simulink model "MPG_MG_PLL_orig"  (R2021b)
settings: Solver=VariableStepAuto  StartTime=0.0  StopTime=1  RelTol=1e-3
model workspace (MAT data in the model file):
  Ts : Simulink.Parameter (value not decoded)
  secondary_on : Simulink.Parameter (value not decoded)
values from neighbouring files (symbols this model uses):
  A = zeros(4,4)    [MPC_MG_script_raw_dmpc.m]    (also in MPG_MG_July.m = [0 1 1 1; 1 0 0 0; 1 0 0 0; 1 0 0 0]; MPG_MG_freq_script.m = ones(4) - eye(4); Script.m = [0 1 1 1 ; 1 0 1 1 ; 1 1 0 1 ; 1 1 1 0])
  C_f = 50e-6    (= 5e-05)    [Four_DG_MG_PrimaryOnlyScript.m]    (also in MPC_MG_script.m; MPC_MG_script_raw_dmpc.m; MPC_MG_secondary_script.m; MPG_MG_July.m)
  f_c = 5000    [Four_DG_MG_PrimaryOnlyScript.m]    (also in MPC_MG_script.m = 40000; MPC_MG_script_raw_dmpc.m = 40000; MPC_MG_secondary_script.m = 40000; MPG_MG_July.m = 50000)
  kL = 1e-5    (= 1e-05)    [Four_DG_MG_PrimaryOnlyScript.m]    (also in MPC_MG_script.m = 1e-08; MPC_MG_script_raw_dmpc.m = 1e-08; MPC_MG_secondary_script.m = 1e-07; MPG_MG_July.m = 1e-07)
  L_f = 1.35e-3    (= 0.00135)    [Four_DG_MG_PrimaryOnlyScript.m]    (also in MPC_MG_script.m; MPC_MG_script_raw_dmpc.m; MPC_MG_secondary_script.m; MPG_MG_July.m)
  L_in1 = 0.35e-3    (= 0.00035)    [Four_DG_MG_PrimaryOnlyScript.m]    (also in MPC_MG_script.m; MPC_MG_script_raw_dmpc.m; MPC_MG_secondary_script.m; MPG_MG_July.m)
  L_in2 = 0.35e-3    (= 0.00035)    [Four_DG_MG_PrimaryOnlyScript.m]    (also in MPC_MG_script.m; MPC_MG_script_raw_dmpc.m; MPC_MG_secondary_script.m; MPG_MG_July.m)
  L_in4 = 0.35e-3    (= 0.00035)    [Four_DG_MG_PrimaryOnlyScript.m]    (also in MPC_MG_script.m; MPC_MG_script_raw_dmpc.m; MPC_MG_secondary_script.m; MPG_MG_July.m)
  lambda1 = [30000 50000 90000 50000]'    [MPC_MG_script_raw_dmpc.m]    (also in MPG_MG_July.m = [4 4 4 4]'; MPG_MG_freq_script.m = [3 3 3 3]'; Script.m = [1 1 1 1]')
  lambda2 = [5 6 7 6]'    [MPC_MG_script_raw_dmpc.m]    (also in MPG_MG_July.m = [0.5e-2 0.5e-2 0.5e-2 0.5e-2]'; MPG_MG_freq_script.m = [1.1 1.9 1.5 1.2]'; Script.m = [0.8e-2 0.8e-2 0.8e-2 0.8e-2]')
  lambda3 = [80000 80000 900000 80000]'    [MPC_MG_script_raw_dmpc.m]    (also in MPG_MG_July.m = [1e-3 1e-3 1e-3 1e-3]'; MPG_MG_freq_script.m = [9e-4 1.2e-2 3e-3 3e-3]'; Script.m = [1.5e-3 1.5e-3 1.5e-3 1.5e-3]')
  LD_ref1 = 800e-6    (= 0.0008)    [Four_DG_MG_PrimaryOnlyScript.m]    (also in MPC_MG_script.m = 0.0003; MPC_MG_script_raw_dmpc.m = 0.0003; MPC_MG_secondary_script.m = 0.0001; MPG_MG_July.m = 0.0004)
  lo_co = 0.2    [Four_DG_MG_PrimaryOnlyScript.m]    (also in MPC_MG_script.m = 0.05; MPC_MG_script_raw_dmpc.m; MPC_MG_secondary_script.m = 0.08; MPG_MG_July.m = 0.15)
  m_p1 = 9.4e-5/droopDivide    (= 9.4e-05)    [Four_DG_MG_PrimaryOnlyScript.m]    (also in MPC_MG_script.m; MPC_MG_script_raw_dmpc.m; MPC_MG_secondary_script.m; MPG_MG_July.m)
  m_p2 = 9.4e-5/droopDivide    (= 9.4e-05)    [Four_DG_MG_PrimaryOnlyScript.m]    (also in MPC_MG_script.m; MPC_MG_script_raw_dmpc.m; MPC_MG_secondary_script.m; MPG_MG_July.m)
  m_p3 = 12.5e-5/droopDivide    (= 0.000125)    [Four_DG_MG_PrimaryOnlyScript.m]    (also in MPC_MG_script.m; MPC_MG_script_raw_dmpc.m; MPC_MG_secondary_script.m; MPG_MG_July.m)
  m_p4 = 12.5e-5/droopDivide    (= 0.000125)    [Four_DG_MG_PrimaryOnlyScript.m]    (also in MPC_MG_script.m; MPC_MG_script_raw_dmpc.m; MPC_MG_secondary_script.m; MPG_MG_July.m)
  N = 3    [MPG_MG_July.m]    (also in MPG_MG_freq_script.m = 2; Script.m = 5)
  n_q1 = 1.3e-3/droopDivide2    (= 0.00013)    [Four_DG_MG_PrimaryOnlyScript.m]    (also in MPC_MG_script.m; MPC_MG_script_raw_dmpc.m; MPC_MG_secondary_script.m; MPG_MG_July.m)
  n_q2 = 1.3e-3/droopDivide2    (= 0.00013)    [Four_DG_MG_PrimaryOnlyScript.m]    (also in MPC_MG_script.m; MPC_MG_script_raw_dmpc.m; MPC_MG_secondary_script.m; MPG_MG_July.m)
  n_q4 = 1.5e-3/droopDivide2    (= 0.00015)    [Four_DG_MG_PrimaryOnlyScript.m]    (also in MPC_MG_script.m; MPC_MG_script_raw_dmpc.m; MPC_MG_secondary_script.m; MPG_MG_July.m)
  Pmax = [45e3 45e3 37e3 37e3]'    [MPG_MG_July.m]    (also in MPG_MG_freq_script.m; Script.m)
  R_f = 0.1    [Four_DG_MG_PrimaryOnlyScript.m]    (also in MPC_MG_script.m; MPC_MG_script_raw_dmpc.m; MPC_MG_secondary_script.m; MPG_MG_July.m)
  R_in1 = 0.03    [Four_DG_MG_PrimaryOnlyScript.m]    (also in MPC_MG_script.m; MPC_MG_script_raw_dmpc.m; MPC_MG_secondary_script.m; MPG_MG_July.m)
  R_in2 = 0.03    [Four_DG_MG_PrimaryOnlyScript.m]    (also in MPC_MG_script.m; MPC_MG_script_raw_dmpc.m; MPC_MG_secondary_script.m; MPG_MG_July.m)
  R_in4 = 0.03    [Four_DG_MG_PrimaryOnlyScript.m]    (also in MPC_MG_script.m; MPC_MG_script_raw_dmpc.m; MPC_MG_secondary_script.m; MPG_MG_July.m)
  time_thresh = 0.6    [Four_DG_MG_PrimaryOnlyScript.m]    (also in MPC_MG_script_raw_dmpc.m = 1.5; MPC_MG_secondary_script.m = 2; MPG_MG_July.m = 0.5; MPG_MG_freq_script.m = 0.5)
  Ts = 10e-6    (= 1e-05)    [Four_DG_MG_PrimaryOnlyScript.m]    (also in MPC_MG_script.m; MPC_MG_script_raw_dmpc.m; MPC_MG_secondary_script.m; MPG_MG_July.m)
  Tsamp = 0.1    [MPG_MG_July.m]    (also in MPG_MG_freq_script.m; Script.m)
  V_nom = 220*sqrt(2)    [Four_DG_MG_PrimaryOnlyScript.m]    (also in MPC_MG_script.m; MPC_MG_script_raw_dmpc.m; MPC_MG_secondary_script.m; MPG_MG_July.m)
  Vdc = 600    [Four_DG_MG_PrimaryOnlyScript.m]    (also in MPC_MG_script.m; MPC_MG_script_raw_dmpc.m; MPC_MG_secondary_script.m; MPG_MG_July.m)
  w_c_high = 2*pi*50    (= 314.159265359)    [Four_DG_MG_PrimaryOnlyScript.m]    (also in MPC_MG_script.m; MPC_MG_script_raw_dmpc.m; MPC_MG_secondary_script.m; MPG_MG_July.m)
  w_nom = 2*pi*50    (= 314.159265359)    [Four_DG_MG_PrimaryOnlyScript.m]    (also in MPC_MG_script.m; MPC_MG_script_raw_dmpc.m; MPC_MG_secondary_script.m; MPG_MG_July.m)
undefined symbols (not defined in the file or in its folder): i
libraries: spsThreePhaseSeriesRLCBranchLib x18, spsabctodq0Lib x16, spsThreePhaseVIMeasurementLib x15, eeGeneralControl x15, dspswit3 x5, spsDCVoltageSourceLib x5, spsSeriesRLCBranchLib x5, spsTwoLevelConverterLib x5, slpidlib x5, spsAlphaBetaZerotodq0Lib x4, spsSecondOrderFilterLib x4, spsThreePhaseSeriesRLCLoadLib x2
(part 4 of 6)

== system MPG_MG_PLL_orig/Voltage Source Inverter 3/Pll1phase/TienXuly ==
  v : Inport
  Gain : Gain  Gain=k
  Integrator : Integrator
  Integrator1 : Integrator
  Locthongthap : TransferFcn  Denominator=[1/fc2 1]
  Mux : Mux  Inputs=2
  Product : Product  RndMeth=Zero
  Product1 : Product  RndMeth=Zero
  Sum : Sum  Inputs=|+-
  Sum1 : Sum  Inputs=|+-
  Sum2 : Sum  Inputs=|+-
  v'-qv' : Scope
  wloc : Constant  Value=fc1*2*pi
  v' : Outport  VectorParamsAs1DForOutWhenUnconnected=off
  v'q : Outport  Port=2  VectorParamsAs1DForOutWhenUnconnected=off
  wires:
  Sum/1 -> Gain/1
  Gain/1 -> Sum1/1, Locthongthap/1
  Sum1/1 -> Product/1
  wloc/1 -> Product/2, Product1/1
  Product/1 -> Integrator/1
  Product1/1 -> Integrator1/1
  Integrator1/1 -> Sum1/2, Sum2/1
  Integrator/1 -> Product1/2, Sum/2, Mux/2, v'/1
  Locthongthap/1 -> Sum2/2
  v/1 -> Sum/1
  Sum2/1 -> v'q/1, Mux/1
  Mux/1 -> v'-qv'/1

== system MPG_MG_PLL_orig/Voltage Source Inverter 3/Pll1phase/apha-beta=>dq ==
  Theta : Inport
  Uapha : Inport  Port=2
  Ubeta : Inport  Port=3
  Mux : Mux  Inputs=3
  Tinhvd : Fcn  Expr=(u[2]*cos(u[1])+u[3]*sin(u[1]))
  Tinhvq : Fcn  Expr=(-u[2]*sin(u[1])+u[3]*cos(u[1]))
  vq : Outport  VectorParamsAs1DForOutWhenUnconnected=off
  vd : Outport  Port=2  VectorParamsAs1DForOutWhenUnconnected=off
  wires:
  Theta/1 -> Mux/1
  Uapha/1 -> Mux/2
  Ubeta/1 -> Mux/3
  Mux/1 -> Tinhvd/1, Tinhvq/1
  Tinhvd/1 -> vd/1
  Tinhvq/1 -> vq/1

== system MPG_MG_PLL_orig/Voltage Source Inverter 3/dq converter/Subsystem ==
  abc : Inport
  wt : Inport  Port=2
  Demux : Demux  Outputs=3
  abc to dq0 : spsabctodq0Lib/abc to dq0  Alignment=90 degrees behind phase A axis
  Out1 : Outport
  Out2 : Outport  Port=2
  wires:
  Demux/1 -> Out1/1
  abc to dq0/1 -> Demux/1
  wt/1 -> abc to dq0/2
  Demux/2 -> Out2/1
  abc/1 -> abc to dq0/1

== system MPG_MG_PLL_orig/Voltage Source Inverter 3/dq converter/Subsystem1 ==
  abc : Inport
  wt : Inport  Port=2
  Demux : Demux  Outputs=3
  abc to dq0 : spsabctodq0Lib/abc to dq0  Alignment=90 degrees behind phase A axis
  Out1 : Outport
  Out2 : Outport  Port=2
  wires:
  Demux/1 -> Out1/1
  abc to dq0/1 -> Demux/1
  wt/1 -> abc to dq0/2
  Demux/2 -> Out2/1
  abc/1 -> abc to dq0/1

== system MPG_MG_PLL_orig/Voltage Source Inverter 3/dq converter/Subsystem2 ==
  abc : Inport
  wt : Inport  Port=2
  Demux : Demux  Outputs=3
  abc to dq0 : spsabctodq0Lib/abc to dq0  Alignment=90 degrees behind phase A axis
  Out1 : Outport
  Out2 : Outport  Port=2
  wires:
  Demux/1 -> Out1/1
  abc to dq0/1 -> Demux/1
  wt/1 -> abc to dq0/2
  Demux/2 -> Out2/1
  abc/1 -> abc to dq0/1

== system MPG_MG_PLL_orig/Voltage Source Inverter 4/CDSC-PLL/DSC16 ==
  Alpha : Inport
  Beta : Inport  Port=2
  DSC_Beta : Subsystem
  DSC_alpha : Subsystem
  DSC2_alp : Outport  VectorParamsAs1DForOutWhenUnconnected=off
  DSC2_Bet : Outport  Port=2  VectorParamsAs1DForOutWhenUnconnected=off
  wires:
  Beta/1 -> DSC_Beta/2(Beta), DSC_alpha/2(Beta)
  Alpha/1 -> DSC_alpha/1(Alpha), DSC_Beta/1(Alpha)
  DSC_Beta/1(Out) -> DSC2_Bet/1
  DSC_alpha/1(Out) -> DSC2_alp/1

== system MPG_MG_PLL_orig/Voltage Source Inverter 4/CDSC-PLL/DSC2 ==
  Alpha : Inport
  Beta : Inport  Port=2
  DSC_Beta : Subsystem
  DSC_alpha : Subsystem
  DSC2_alp : Outport  VectorParamsAs1DForOutWhenUnconnected=off
  DSC2_Bet : Outport  Port=2  VectorParamsAs1DForOutWhenUnconnected=off
  wires:
  DSC_alpha/1(Out) -> DSC2_alp/1
  DSC_Beta/1(Out) -> DSC2_Bet/1
  Alpha/1 -> DSC_Beta/1(Alpha), DSC_alpha/1(Alpha)
  Beta/1 -> DSC_alpha/2(Beta), DSC_Beta/2(Beta)

== system MPG_MG_PLL_orig/Voltage Source Inverter 4/CDSC-PLL/DSC4 ==
  Alpha : Inport
  Beta : Inport  Port=2
  DSC_Beta : Subsystem
  DSC_alpha : Subsystem
  DSC2_alp : Outport  VectorParamsAs1DForOutWhenUnconnected=off
  DSC2_Bet : Outport  Port=2  VectorParamsAs1DForOutWhenUnconnected=off
  wires:
  Beta/1 -> DSC_Beta/2(Beta), DSC_alpha/2(Beta)
  Alpha/1 -> DSC_alpha/1(Alpha), DSC_Beta/1(Alpha)
  DSC_Beta/1(Out) -> DSC2_Bet/1
  DSC_alpha/1(Out) -> DSC2_alp/1

== system MPG_MG_PLL_orig/Voltage Source Inverter 4/CDSC-PLL/DSC8 ==
  Alpha : Inport
  Beta : Inport  Port=2
  DSC_Beta : Subsystem
  DSC_alpha : Subsystem
  DSC2_alp : Outport  VectorParamsAs1DForOutWhenUnconnected=off
  DSC2_Bet : Outport  Port=2  VectorParamsAs1DForOutWhenUnconnected=off
  wires:
  DSC_alpha/1(Out) -> DSC2_alp/1
  DSC_Beta/1(Out) -> DSC2_Bet/1
  Alpha/1 -> DSC_Beta/1(Alpha), DSC_alpha/1(Alpha)
  Beta/1 -> DSC_alpha/2(Beta), DSC_Beta/2(Beta)

== system MPG_MG_PLL_orig/Voltage Source Inverter 4/CDSC-PLL/SRF-PLL1 ==
  al-be-0 : Inport
  1/2/pi : Gain  Gain=1/(2*pi)
  2 : Constant  Value=2*pi
  3 : Constant  Value=0
  Al_Be_0 to dq0 : Subsystem
      mask Display:
      | plot([0 1], [0,1])
      | port_label('input', 1, '\alpha\beta0','texmode','on')
      | port_label('input', 2, 'wt')
      | port_label('output', 1, 'dq0')
  Integrator : Integrator
  Math Function : Math  Operator=mod  SignedPower=on  SaturateOnIntegerOverflow=on
  "PI " : slpidlib/PID Controller  Controller=PI  Form=Parallel  TimeDomain=Continuous-time  UseExternalTs=off  SampleTime=100e-6  IntegratorMethod=Forward Euler  FilterMethod=Forward Euler  ControllerParametersSource=internal  P=10  I=30  D=0  UseFilter=on  N=100  TunerSelectOption=Transfer Function Based (PID Tuner App)  InitialConditionSource=internal  InitialConditionForIntegrator=0  InitialConditionForFilter=0  DifferentiatorICPrevScaledInput=0  ExternalReset=none  TrackingMode=off  Kt=1  LimitOutput=off  SatLimitsSource=internal  UpperSaturationLimit=inf  LowerSaturationLimit=-inf  LinearizeAsGain=on  AntiWindupMode=none  Kb=1  POutMin=[]  POutMax=[]  IOutMin=[]  IOutMax=[]  DOutMin=[]  DOutMax=[]  NOutMin=[]  NOutMax=[]  SumOutMin=[]  SumOutMax=[]  SaturationOutMin=[]  SaturationOutMax=[]  PParamMin=[]  PParamMax=[]  IParamMin=[]  IParamMax=[]  DParamMin=[]  DParamMax=[]  NParamMin=[]  NParamMax=[]  KbParamMin=[]  KbParamMax=[]  KtParamMin=[]  KtParamMax=[]  KbOutMin=[]  KbOutMax=[]  KtOutMin=[]  KtOutMax=[]  IntegratorOutMin=[]  IntegratorOutMax=[]  FilterOutMin=[]  FilterOutMax=[]  SumI1OutMin=[]  SumI1OutMax=[]  SumI2OutMin=[]  SumI2OutMax=[]  SumI3OutMin=[]  SumI3OutMax=[]  SumI4OutMin=[]  SumI4OutMax=[]  SumDOutMin=[]  SumDOutMax=[]  DifferentiatorOutMin=[]  DifferentiatorOutMax=[]  FilterDiffOutCoefMin=[]  FilterDiffOutCoefMax=[]  ReciprocalOutMin=[]  ReciprocalOutMax=[]  SumDenOutMin=[]  SumDenOutMax=[]  SumNumOutMin=[]  SumNumOutMax=[]  DivideOutMin=[]  DivideOutMax=[]  UdiffTsProdOutMin=[]  UdiffTsProdOutMax=[]  NTsProdOutMin=[]  NTsProdOutMax=[]  UintegralTsProdOutMin=[]  UintegralTsProdOutMax=[]  UngainTsProdOutMin=[]  UngainTsProdOutMax=[]  IntegratorContinuousStateAttributes=''  IntegratorStateMustResolveToSignalObject=off  IntegratorRTWStateStorageClass=Auto  FilterContinuousStateAttributes=''  FilterStateMustResolveToSignalObject=off  FilterRTWStateStorageClass=Auto  ParallelPVariant=InternalParameters  IdealPVariant=Disabled  IVariant=InternalParameters  DVariant=Disabled  IntegratorVariant=Continuous  SatVariant=Disabled  AWVariant=Passthrough  PCopyVariant=Disabled  TRVariant=Disabled  FdbkBlocksVariant=Forward  IdealPFdbkVariant=Disabled  SatFdbkVariant=Disabled  DerivativeFilterVariant=Disabled  NVariant=Disabled  NCopyVariant=Disabled_SignalSpec  FilterICVariant=Disabled  IntegratorICVariant=InternalICs  ExternalResetVariant=Disabled  TRSumVariant=Passthrough  SumFdbkVariant=Disabled  SumVariant=Sum_PI  TsampFilterVariant=InternalTs  TsampNgainVariant=Passthrough  TsampIntegralVariant=Passthrough  ExternalSaturationOutDataTypeStr=Inherit: Same as second input
  Scope2 : Scope  NumInputPorts=2
  Second-Order Filter : spsSecondOrderFilterLib/Second-Order Filter  FilterType=Lowpass  Fo=5  Zeta=0.707  Ts=0  Initialize=off  Vac_Init="[0,  0,  50]"  Vdc_Init=0  PlotResponse=off  FreqRange=[0, 500, 1]
      settings: SourceProductBaseCode=PS
  Selector : Selector  InputPortWidth=3  IndexOptions=Index vector (dialog)  Indices=1  OutputSizes=1
  Sum1 : Sum  Inputs=|++
  Sum2 : Sum  Inputs=|+-
  w : Constant  Value=100*pi
  f : Outport  VectorParamsAs1DForOutWhenUnconnected=off
  wt : Outport  Port=2  VectorParamsAs1DForOutWhenUnconnected=off
  wires:
  1/2/pi/1 -> Second-Order Filter/1, Scope2/2
  Math Function/1 -> Al_Be_0 to dq0/2(wt), wt/1
  Integrator/1 -> Math Function/1
  2/1 -> Math Function/2
  Sum1/1 -> Integrator/1, 1/2/pi/1
  w/1 -> Sum1/2
  "PI "/1 -> Sum1/1
  Sum2/1 -> "PI "/1
  al-be-0/1 -> Al_Be_0 to dq0/1(Al_Be_0)
  3/1 -> Sum2/2
  Al_Be_0 to dq0/1(dq0) -> Selector/1
  Selector/1 -> Sum2/1, Scope2/1
  Second-Order Filter/1 -> f/1

== system MPG_MG_PLL_orig/Voltage Source Inverter 4/CDSC-PLL/abc to alpha-beta-Zero ==
  abc : Inport
  Gain1 : Gain  Gain=(2/3)  SaturateOnIntegerOverflow=on  OutDataTypeStr=Inherit: Same as input  ParamDataTypeStr=Inherit: Same as input
  Gain3 : Gain  Gain="[ 1   -1/2   -1/2; 0   sqrt(3)/2   -sqrt(3)/2; 1/(2)  1/(2)  1/(2) ]"  Multiplication=Matrix(K*u) (u vector)  SaturateOnIntegerOverflow=on  OutDataTypeStr=Inherit: Same as input  ParamDataTypeStr=Inherit: Same as input
  al_be_0 : Outport  VectorParamsAs1DForOutWhenUnconnected=off
  wires:
  Gain3/1 -> Gain1/1
  Gain1/1 -> al_be_0/1
  abc/1 -> Gain3/1

== system MPG_MG_PLL_orig/Voltage Source Inverter 4/dq converter/Subsystem ==
  abc : Inport
  wt : Inport  Port=2
  Demux : Demux  Outputs=3
  abc to dq0 : spsabctodq0Lib/abc to dq0  Alignment=90 degrees behind phase A axis
  Out1 : Outport
  Out2 : Outport  Port=2
  wires:
  Demux/1 -> Out1/1
  abc to dq0/1 -> Demux/1
  wt/1 -> abc to dq0/2
  Demux/2 -> Out2/1
  abc/1 -> abc to dq0/1

== system MPG_MG_PLL_orig/Voltage Source Inverter 4/dq converter/Subsystem1 ==
  abc : Inport
  wt : Inport  Port=2
  Demux : Demux  Outputs=3
  abc to dq0 : spsabctodq0Lib/abc to dq0  Alignment=90 degrees behind phase A axis
  Out1 : Outport
  Out2 : Outport  Port=2
  wires:
  Demux/1 -> Out1/1
  abc to dq0/1 -> Demux/1
  wt/1 -> abc to dq0/2
  Demux/2 -> Out2/1
  abc/1 -> abc to dq0/1

== system MPG_MG_PLL_orig/Voltage Source Inverter 4/dq converter/Subsystem2 ==
  abc : Inport
  wt : Inport  Port=2
  Demux : Demux  Outputs=3
  abc to dq0 : spsabctodq0Lib/abc to dq0  Alignment=90 degrees behind phase A axis
  Out1 : Outport
  Out2 : Outport  Port=2
  wires:
  Demux/1 -> Out1/1
  abc to dq0/1 -> Demux/1
  wt/1 -> abc to dq0/2
  Demux/2 -> Out2/1
  abc/1 -> abc to dq0/1

== system MPG_MG_PLL_orig/Voltage Source Inverter 5/CDSC-PLL/DSC16 ==
  Alpha : Inport
  Beta : Inport  Port=2
  DSC_Beta : Subsystem
  DSC_alpha : Subsystem
  DSC2_alp : Outport  VectorParamsAs1DForOutWhenUnconnected=off
  DSC2_Bet : Outport  Port=2  VectorParamsAs1DForOutWhenUnconnected=off
  wires:
  Beta/1 -> DSC_Beta/2(Beta), DSC_alpha/2(Beta)
  Alpha/1 -> DSC_alpha/1(Alpha), DSC_Beta/1(Alpha)
  DSC_Beta/1(Out) -> DSC2_Bet/1
  DSC_alpha/1(Out) -> DSC2_alp/1

== system MPG_MG_PLL_orig/Voltage Source Inverter 5/CDSC-PLL/DSC2 ==
  Alpha : Inport
  Beta : Inport  Port=2
  DSC_Beta : Subsystem
  DSC_alpha : Subsystem
  DSC2_alp : Outport  VectorParamsAs1DForOutWhenUnconnected=off
  DSC2_Bet : Outport  Port=2  VectorParamsAs1DForOutWhenUnconnected=off
  wires:
  DSC_alpha/1(Out) -> DSC2_alp/1
  DSC_Beta/1(Out) -> DSC2_Bet/1
  Alpha/1 -> DSC_Beta/1(Alpha), DSC_alpha/1(Alpha)
  Beta/1 -> DSC_alpha/2(Beta), DSC_Beta/2(Beta)

== system MPG_MG_PLL_orig/Voltage Source Inverter 5/CDSC-PLL/DSC4 ==
  Alpha : Inport
  Beta : Inport  Port=2
  DSC_Beta : Subsystem
  DSC_alpha : Subsystem
  DSC2_alp : Outport  VectorParamsAs1DForOutWhenUnconnected=off
  DSC2_Bet : Outport  Port=2  VectorParamsAs1DForOutWhenUnconnected=off
  wires:
  Beta/1 -> DSC_Beta/2(Beta), DSC_alpha/2(Beta)
  Alpha/1 -> DSC_alpha/1(Alpha), DSC_Beta/1(Alpha)
  DSC_Beta/1(Out) -> DSC2_Bet/1
  DSC_alpha/1(Out) -> DSC2_alp/1

== system MPG_MG_PLL_orig/Voltage Source Inverter 5/CDSC-PLL/DSC8 ==
  Alpha : Inport
  Beta : Inport  Port=2
  DSC_Beta : Subsystem
  DSC_alpha : Subsystem
  DSC2_alp : Outport  VectorParamsAs1DForOutWhenUnconnected=off
  DSC2_Bet : Outport  Port=2  VectorParamsAs1DForOutWhenUnconnected=off
  wires:
  DSC_alpha/1(Out) -> DSC2_alp/1
  DSC_Beta/1(Out) -> DSC2_Bet/1
  Alpha/1 -> DSC_Beta/1(Alpha), DSC_alpha/1(Alpha)
  Beta/1 -> DSC_alpha/2(Beta), DSC_Beta/2(Beta)

== system MPG_MG_PLL_orig/Voltage Source Inverter 5/CDSC-PLL/SRF-PLL1 ==
  al-be-0 : Inport
  1/2/pi : Gain  Gain=1/(2*pi)
  2 : Constant  Value=2*pi
  3 : Constant  Value=0
  Al_Be_0 to dq0 : Subsystem
      mask Display:
      | plot([0 1], [0,1])
      | port_label('input', 1, '\alpha\beta0','texmode','on')
      | port_label('input', 2, 'wt')
      | port_label('output', 1, 'dq0')
  Integrator : Integrator
  Math Function : Math  Operator=mod  SignedPower=on  SaturateOnIntegerOverflow=on
  "PI " : slpidlib/PID Controller  Controller=PI  Form=Parallel  TimeDomain=Continuous-time  UseExternalTs=off  SampleTime=100e-6  IntegratorMethod=Forward Euler  FilterMethod=Forward Euler  ControllerParametersSource=internal  P=10  I=30  D=0  UseFilter=on  N=100  TunerSelectOption=Transfer Function Based (PID Tuner App)  InitialConditionSource=internal  InitialConditionForIntegrator=0  InitialConditionForFilter=0  DifferentiatorICPrevScaledInput=0  ExternalReset=none  TrackingMode=off  Kt=1  LimitOutput=off  SatLimitsSource=internal  UpperSaturationLimit=inf  LowerSaturationLimit=-inf  LinearizeAsGain=on  AntiWindupMode=none  Kb=1  POutMin=[]  POutMax=[]  IOutMin=[]  IOutMax=[]  DOutMin=[]  DOutMax=[]  NOutMin=[]  NOutMax=[]  SumOutMin=[]  SumOutMax=[]  SaturationOutMin=[]  SaturationOutMax=[]  PParamMin=[]  PParamMax=[]  IParamMin=[]  IParamMax=[]  DParamMin=[]  DParamMax=[]  NParamMin=[]  NParamMax=[]  KbParamMin=[]  KbParamMax=[]  KtParamMin=[]  KtParamMax=[]  KbOutMin=[]  KbOutMax=[]  KtOutMin=[]  KtOutMax=[]  IntegratorOutMin=[]  IntegratorOutMax=[]  FilterOutMin=[]  FilterOutMax=[]  SumI1OutMin=[]  SumI1OutMax=[]  SumI2OutMin=[]  SumI2OutMax=[]  SumI3OutMin=[]  SumI3OutMax=[]  SumI4OutMin=[]  SumI4OutMax=[]  SumDOutMin=[]  SumDOutMax=[]  DifferentiatorOutMin=[]  DifferentiatorOutMax=[]  FilterDiffOutCoefMin=[]  FilterDiffOutCoefMax=[]  ReciprocalOutMin=[]  ReciprocalOutMax=[]  SumDenOutMin=[]  SumDenOutMax=[]  SumNumOutMin=[]  SumNumOutMax=[]  DivideOutMin=[]  DivideOutMax=[]  UdiffTsProdOutMin=[]  UdiffTsProdOutMax=[]  NTsProdOutMin=[]  NTsProdOutMax=[]  UintegralTsProdOutMin=[]  UintegralTsProdOutMax=[]  UngainTsProdOutMin=[]  UngainTsProdOutMax=[]  IntegratorContinuousStateAttributes=''  IntegratorStateMustResolveToSignalObject=off  IntegratorRTWStateStorageClass=Auto  FilterContinuousStateAttributes=''  FilterStateMustResolveToSignalObject=off  FilterRTWStateStorageClass=Auto  ParallelPVariant=InternalParameters  IdealPVariant=Disabled  IVariant=InternalParameters  DVariant=Disabled  IntegratorVariant=Continuous  SatVariant=Disabled  AWVariant=Passthrough  PCopyVariant=Disabled  TRVariant=Disabled  FdbkBlocksVariant=Forward  IdealPFdbkVariant=Disabled  SatFdbkVariant=Disabled  DerivativeFilterVariant=Disabled  NVariant=Disabled  NCopyVariant=Disabled_SignalSpec  FilterICVariant=Disabled  IntegratorICVariant=InternalICs  ExternalResetVariant=Disabled  TRSumVariant=Passthrough  SumFdbkVariant=Disabled  SumVariant=Sum_PI  TsampFilterVariant=InternalTs  TsampNgainVariant=Passthrough  TsampIntegralVariant=Passthrough  ExternalSaturationOutDataTypeStr=Inherit: Same as second input
  Scope2 : Scope  NumInputPorts=2
  Second-Order Filter : spsSecondOrderFilterLib/Second-Order Filter  FilterType=Lowpass  Fo=5  Zeta=0.707  Ts=0  Initialize=off  Vac_Init="[0,  0,  50]"  Vdc_Init=0  PlotResponse=off  FreqRange=[0, 500, 1]
      settings: SourceProductBaseCode=PS
  Selector : Selector  InputPortWidth=3  IndexOptions=Index vector (dialog)  Indices=1  OutputSizes=1
  Sum1 : Sum  Inputs=|++
  Sum2 : Sum  Inputs=|+-
  w : Constant  Value=100*pi
  f : Outport  VectorParamsAs1DForOutWhenUnconnected=off
  wt : Outport  Port=2  VectorParamsAs1DForOutWhenUnconnected=off
  wires:
  1/2/pi/1 -> Second-Order Filter/1, Scope2/2
  Math Function/1 -> Al_Be_0 to dq0/2(wt), wt/1
  Integrator/1 -> Math Function/1
  2/1 -> Math Function/2
  Sum1/1 -> Integrator/1, 1/2/pi/1
  w/1 -> Sum1/2
  "PI "/1 -> Sum1/1
  Sum2/1 -> "PI "/1
  al-be-0/1 -> Al_Be_0 to dq0/1(Al_Be_0)
  3/1 -> Sum2/2
  Al_Be_0 to dq0/1(dq0) -> Selector/1
  Selector/1 -> Sum2/1, Scope2/1
  Second-Order Filter/1 -> f/1

== system MPG_MG_PLL_orig/Voltage Source Inverter 5/CDSC-PLL/abc to alpha-beta-Zero ==
  abc : Inport
  Gain1 : Gain  Gain=(2/3)  SaturateOnIntegerOverflow=on  OutDataTypeStr=Inherit: Same as input  ParamDataTypeStr=Inherit: Same as input
  Gain3 : Gain  Gain="[ 1   -1/2   -1/2; 0   sqrt(3)/2   -sqrt(3)/2; 1/(2)  1/(2)  1/(2) ]"  Multiplication=Matrix(K*u) (u vector)  SaturateOnIntegerOverflow=on  OutDataTypeStr=Inherit: Same as input  ParamDataTypeStr=Inherit: Same as input
  al_be_0 : Outport  VectorParamsAs1DForOutWhenUnconnected=off
  wires:
  Gain3/1 -> Gain1/1
  Gain1/1 -> al_be_0/1
  abc/1 -> Gain3/1

== system MPG_MG_PLL_orig/Voltage Source Inverter 5/dq converter/Subsystem ==
  abc : Inport
  wt : Inport  Port=2
  Demux : Demux  Outputs=3
  abc to dq0 : spsabctodq0Lib/abc to dq0  Alignment=90 degrees behind phase A axis
  Out1 : Outport
  Out2 : Outport  Port=2
  wires:
  Demux/1 -> Out1/1
  abc to dq0/1 -> Demux/1
  wt/1 -> abc to dq0/2
  Demux/2 -> Out2/1
  abc/1 -> abc to dq0/1

== system MPG_MG_PLL_orig/Voltage Source Inverter 5/dq converter/Subsystem1 ==
  abc : Inport
  wt : Inport  Port=2
  Demux : Demux  Outputs=3
  abc to dq0 : spsabctodq0Lib/abc to dq0  Alignment=90 degrees behind phase A axis
  Out1 : Outport
  Out2 : Outport  Port=2
  wires:
  Demux/1 -> Out1/1
  abc to dq0/1 -> Demux/1
  wt/1 -> abc to dq0/2
  Demux/2 -> Out2/1
  abc/1 -> abc to dq0/1

== system MPG_MG_PLL_orig/Voltage Source Inverter 5/dq converter/Subsystem2 ==
  abc : Inport
  wt : Inport  Port=2
  Demux : Demux  Outputs=3
  abc to dq0 : spsabctodq0Lib/abc to dq0  Alignment=90 degrees behind phase A axis
  Out1 : Outport
  Out2 : Outport  Port=2
  wires:
  Demux/1 -> Out1/1
  abc to dq0/1 -> Demux/1
  wt/1 -> abc to dq0/2
  Demux/2 -> Out2/1
  abc/1 -> abc to dq0/1

== system MPG_MG_PLL_orig/Voltage Source Inverter 2/CDSC-PLL/DSC16/DSC_Beta ==
  Alpha : Inport
  Beta : Inport  Port=2
  Cos 2*pi/n : Subsystem
  Divide : Product  Inputs=*/
  Divide1 : Product  Inputs=*/
  Gain : Gain  Gain=1/2
  Product : Product
  Product1 : Product
  Sin 2*pi/n : Subsystem
  Sum1 : Sum  Inputs=+++
  T/n : Constant  Value=1/n
  T/n1 : Constant  Value=1/n
  Variable Transport Delay : VariableTransportDelay  VariableDelayType=Variable transport delay  MaximumDelay=10
  Variable Transport Delay1 : VariableTransportDelay  VariableDelayType=Variable transport delay  MaximumDelay=10
  Out : Outport  VectorParamsAs1DForOutWhenUnconnected=off
  wires:
  Gain/1 -> Out/1
  Sum1/1 -> Gain/1
  Beta/1 -> Variable Transport Delay/1, Sum1/1
  Alpha/1 -> Variable Transport Delay1/1
  Cos 2*pi/n/1(cos) -> Product/2
  Product/1 -> Sum1/2
  Variable Transport Delay/1 -> Product/1
  Variable Transport Delay1/1 -> Product1/1
  Product1/1 -> Sum1/3
  Sin 2*pi/n/1(sin) -> Product1/2
  T/n/1 -> Divide/1
  Divide/1 -> Variable Transport Delay/2
  [f_pll_c3] -> Divide/2
  T/n1/1 -> Divide1/1
  Divide1/1 -> Variable Transport Delay1/2
  [f_pll_c3] -> Divide1/2

== system MPG_MG_PLL_orig/Voltage Source Inverter 2/CDSC-PLL/DSC16/DSC_alpha ==
  Alpha : Inport
  Beta : Inport  Port=2
  Cos 2*pi/n : Subsystem
  Divide : Product  Inputs=*/
  Divide1 : Product  Inputs=*/
  Gain : Gain  Gain=1/2
  Product : Product
  Product1 : Product
  Sin 2*pi/n : Subsystem
  Sum1 : Sum  Inputs=++-
  T/n : Constant  Value=1/n
  T/n1 : Constant  Value=1/n
  Variable Transport Delay : VariableTransportDelay  VariableDelayType=Variable transport delay  MaximumDelay=10
  Variable Transport Delay1 : VariableTransportDelay  VariableDelayType=Variable transport delay  MaximumDelay=10
  Out : Outport  VectorParamsAs1DForOutWhenUnconnected=off
  wires:
  Sum1/1 -> Gain/1
  Gain/1 -> Out/1
  Sin 2*pi/n/1(sin) -> Product1/2
  Beta/1 -> Variable Transport Delay1/1
  Product1/1 -> Sum1/3
  Variable Transport Delay1/1 -> Product1/1
  Alpha/1 -> Variable Transport Delay/1, Sum1/1
  Variable Transport Delay/1 -> Product/1
  Product/1 -> Sum1/2
  Cos 2*pi/n/1(cos) -> Product/2
  T/n/1 -> Divide/1
  Divide/1 -> Variable Transport Delay/2
  [f_pll_c3] -> Divide/2
  T/n1/1 -> Divide1/1
  Divide1/1 -> Variable Transport Delay1/2
  [f_pll_c3] -> Divide1/2

== system MPG_MG_PLL_orig/Voltage Source Inverter 2/CDSC-PLL/DSC2/DSC_Beta ==
  Alpha : Inport
  Beta : Inport  Port=2
  Cos 2*pi/n : Subsystem
  Divide : Product  Inputs=*/
  Divide1 : Product  Inputs=*/
  Gain : Gain  Gain=1/2
  Product : Product
  Product1 : Product
  Sin 2*pi/n : Subsystem
  Sum1 : Sum  Inputs=+++
  T/n : Constant  Value=1/n
  T/n1 : Constant  Value=1/n
  Variable Transport Delay : VariableTransportDelay  VariableDelayType=Variable transport delay  MaximumDelay=10
  Variable Transport Delay1 : VariableTransportDelay  VariableDelayType=Variable transport delay  MaximumDelay=10
  Out : Outport  VectorParamsAs1DForOutWhenUnconnected=off
  wires:
  Sin 2*pi/n/1(sin) -> Product1/2
  Product1/1 -> Sum1/3
  Variable Transport Delay1/1 -> Product1/1
  Variable Transport Delay/1 -> Product/1
  Product/1 -> Sum1/2
  Cos 2*pi/n/1(cos) -> Product/2
  Alpha/1 -> Variable Transport Delay1/1
  Beta/1 -> Sum1/1, Variable Transport Delay/1
  Sum1/1 -> Gain/1
  Gain/1 -> Out/1
  T/n1/1 -> Divide/1
  Divide/1 -> Variable Transport Delay1/2
  [f_pll_c3] -> Divide/2
  T/n/1 -> Divide1/1
  Divide1/1 -> Variable Transport Delay/2
  [f_pll_c3] -> Divide1/2

== system MPG_MG_PLL_orig/Voltage Source Inverter 2/CDSC-PLL/DSC2/DSC_alpha ==
  Alpha : Inport
  Beta : Inport  Port=2
  Cos 2*pi/n : Subsystem
  Divide : Product  Inputs=*/
  Divide1 : Product  Inputs=*/
  Gain : Gain  Gain=1/2
  Product : Product
  Product1 : Product
  Sin 2*pi/n : Subsystem
  Sum1 : Sum  Inputs=++-
  T/n : Constant  Value=1/n
  T/n. : Constant  Value=1/n
  Variable Transport Delay : VariableTransportDelay  VariableDelayType=Variable transport delay  MaximumDelay=10
  Variable Transport Delay1 : VariableTransportDelay  VariableDelayType=Variable transport delay  MaximumDelay=10
  Out : Outport  VectorParamsAs1DForOutWhenUnconnected=off
  wires:
  Cos 2*pi/n/1(cos) -> Product/2
  Product/1 -> Sum1/2
  Variable Transport Delay/1 -> Product/1
  Alpha/1 -> Variable Transport Delay/1, Sum1/1
  Variable Transport Delay1/1 -> Product1/1
  Product1/1 -> Sum1/3
  Beta/1 -> Variable Transport Delay1/1
  Sin 2*pi/n/1(sin) -> Product1/2
  Gain/1 -> Out/1
  Sum1/1 -> Gain/1
  T/n/1 -> Divide/1
  Divide/1 -> Variable Transport Delay/2
  [f_pll_c3] -> Divide/2
  Divide1/1 -> Variable Transport Delay1/2
  T/n./1 -> Divide1/1
  [f_pll_c3] -> Divide1/2

== system MPG_MG_PLL_orig/Voltage Source Inverter 2/CDSC-PLL/DSC4/DSC_Beta ==
  Alpha : Inport
  Beta : Inport  Port=2
  Cos 2*pi/n : Subsystem
  Divide : Product  Inputs=*/
  Divide1 : Product  Inputs=*/
  Gain : Gain  Gain=1/2
  Product : Product
  Product1 : Product
  Sin 2*pi/n : Subsystem
  Sum1 : Sum  Inputs=+++
  T/n : Constant  Value=1/n
  T/n1 : Constant  Value=1/n
  Variable Transport Delay : VariableTransportDelay  VariableDelayType=Variable transport delay  MaximumDelay=10
  Variable Transport Delay1 : VariableTransportDelay  VariableDelayType=Variable transport delay  MaximumDelay=10
  Out : Outport  VectorParamsAs1DForOutWhenUnconnected=off
  wires:
  Gain/1 -> Out/1
  Sum1/1 -> Gain/1
  Beta/1 -> Variable Transport Delay/1, Sum1/1
  Alpha/1 -> Variable Transport Delay1/1
  Cos 2*pi/n/1(cos) -> Product/2
  Product/1 -> Sum1/2
  Variable Transport Delay/1 -> Product/1
  Variable Transport Delay1/1 -> Product1/1
  Product1/1 -> Sum1/3
  Sin 2*pi/n/1(sin) -> Product1/2
  T/n/1 -> Divide/1
  Divide/1 -> Variable Transport Delay/2
  [f_pll_c3] -> Divide/2
  T/n1/1 -> Divide1/1
  Divide1/1 -> Variable Transport Delay1/2
  [f_pll_c3] -> Divide1/2

== system MPG_MG_PLL_orig/Voltage Source Inverter 2/CDSC-PLL/DSC4/DSC_alpha ==
  Alpha : Inport
  Beta : Inport  Port=2
  Cos 2*pi/n : Subsystem
  Divide : Product  Inputs=*/
  Divide1 : Product  Inputs=*/
  Gain : Gain  Gain=1/2
  Product : Product
  Product1 : Product
  Sin 2*pi/n : Subsystem
  Sum1 : Sum  Inputs=++-
  T/n : Constant  Value=1/n
  T/n1 : Constant  Value=1/n
  Variable Transport Delay : VariableTransportDelay  VariableDelayType=Variable transport delay  MaximumDelay=10
  Variable Transport Delay1 : VariableTransportDelay  VariableDelayType=Variable transport delay  MaximumDelay=10
  Out : Outport  VectorParamsAs1DForOutWhenUnconnected=off
  wires:
  Sum1/1 -> Gain/1
  Gain/1 -> Out/1
  Sin 2*pi/n/1(sin) -> Product1/2
  Beta/1 -> Variable Transport Delay1/1
  Product1/1 -> Sum1/3
  Variable Transport Delay1/1 -> Product1/1
  Alpha/1 -> Variable Transport Delay/1, Sum1/1
  Variable Transport Delay/1 -> Product/1
  Product/1 -> Sum1/2
  Cos 2*pi/n/1(cos) -> Product/2
  T/n1/1 -> Divide/1
  Divide/1 -> Variable Transport Delay1/2
  [f_pll_c3] -> Divide/2
  T/n/1 -> Divide1/1
  Divide1/1 -> Variable Transport Delay/2
  [f_pll_c3] -> Divide1/2

== system MPG_MG_PLL_orig/Voltage Source Inverter 2/CDSC-PLL/DSC8/DSC_Beta ==
  Alpha : Inport
  Beta : Inport  Port=2
  Cos 2*pi/n : Subsystem
  Divide : Product  Inputs=*/
  Divide1 : Product  Inputs=*/
  Gain : Gain  Gain=1/2
  Product : Product
  Product1 : Product
  Sin 2*pi/n : Subsystem
  Sum1 : Sum  Inputs=+++
  T/n : Constant  Value=1/n
  T/n1 : Constant  Value=1/n
  Variable Transport Delay : VariableTransportDelay  VariableDelayType=Variable transport delay  MaximumDelay=10
  Variable Transport Delay1 : VariableTransportDelay  VariableDelayType=Variable transport delay  MaximumDelay=10
  Out : Outport  VectorParamsAs1DForOutWhenUnconnected=off
  wires:
  Sin 2*pi/n/1(sin) -> Product1/2
  Product1/1 -> Sum1/3
  Variable Transport Delay1/1 -> Product1/1
  Variable Transport Delay/1 -> Product/1
  Product/1 -> Sum1/2
  Cos 2*pi/n/1(cos) -> Product/2
  Alpha/1 -> Variable Transport Delay1/1
  Beta/1 -> Sum1/1, Variable Transport Delay/1
  Sum1/1 -> Gain/1
  Gain/1 -> Out/1
  T/n/1 -> Divide/1
  Divide/1 -> Variable Transport Delay/2
  [f_pll_c3] -> Divide/2
  T/n1/1 -> Divide1/1
  Divide1/1 -> Variable Transport Delay1/2
  [f_pll_c3] -> Divide1/2

== system MPG_MG_PLL_orig/Voltage Source Inverter 2/CDSC-PLL/DSC8/DSC_alpha ==
  Alpha : Inport
  Beta : Inport  Port=2
  Cos 2*pi/n : Subsystem
  Divide : Product  Inputs=*/
  Divide1 : Product  Inputs=*/
  Gain : Gain  Gain=1/2
  Product : Product
  Product1 : Product
  Sin 2*pi/n : Subsystem
  Sum1 : Sum  Inputs=++-
  T/n : Constant  Value=1/n
  T/n1 : Constant  Value=1/n
  Variable Transport Delay : VariableTransportDelay  VariableDelayType=Variable transport delay  MaximumDelay=10
  Variable Transport Delay1 : VariableTransportDelay  VariableDelayType=Variable transport delay  MaximumDelay=10
  Out : Outport  VectorParamsAs1DForOutWhenUnconnected=off
  wires:
  Cos 2*pi/n/1(cos) -> Product/2
  Product/1 -> Sum1/2
  Variable Transport Delay/1 -> Product/1
  Alpha/1 -> Variable Transport Delay/1, Sum1/1
  Variable Transport Delay1/1 -> Product1/1
  Product1/1 -> Sum1/3
  Beta/1 -> Variable Transport Delay1/1
  Sin 2*pi/n/1(sin) -> Product1/2
  Gain/1 -> Out/1
  Sum1/1 -> Gain/1
  T/n/1 -> Divide/1
  Divide/1 -> Variable Transport Delay/2
  [f_pll_c3] -> Divide/2
  T/n1/1 -> Divide1/1
  Divide1/1 -> Variable Transport Delay1/2
  [f_pll_c3] -> Divide1/2

== system MPG_MG_PLL_orig/Voltage Source Inverter 2/CDSC-PLL/SRF-PLL1/Al_Be_0 to dq0 ==
  Al_Be_0 : Inport
  wt : Inport  Port=2
  Fcn : Fcn  Expr=u[1]*cos(u[4]) + u[2]*sin(u[4])
  Fcn1 : Fcn  Expr=-u[1]*sin(u[4]) + u[2]*cos(u[4])
  Fcn2 : Fcn  Expr=u[3]
  Mux1 : Mux  Inputs=[3 1]
  Mux2 : Mux  Inputs=3
  dq0 : Outport  VectorParamsAs1DForOutWhenUnconnected=off
  wires:
  Mux1/1 -> Fcn/1, Fcn2/1, Fcn1/1
  Fcn1/1 -> Mux2/2
  wt/1 -> Mux1/2
  Mux2/1 -> dq0/1
  Al_Be_0/1 -> Mux1/1
  Fcn2/1 -> Mux2/3
  Fcn/1 -> Mux2/1

== system MPG_MG_PLL_orig/Voltage Source Inverter 3/CDSC-PLL/DSC16/DSC_Beta ==
  Alpha : Inport
  Beta : Inport  Port=2
  Cos 2*pi/n : Subsystem
  Divide : Product  Inputs=*/
  Divide1 : Product  Inputs=*/
  Gain : Gain  Gain=1/2
  Product : Product
  Product1 : Product
  Sin 2*pi/n : Subsystem
  Sum1 : Sum  Inputs=+++
  T/n : Constant  Value=1/n
  T/n1 : Constant  Value=1/n
  Variable Transport Delay : VariableTransportDelay  VariableDelayType=Variable transport delay  MaximumDelay=10
  Variable Transport Delay1 : VariableTransportDelay  VariableDelayType=Variable transport delay  MaximumDelay=10
  Out : Outport  VectorParamsAs1DForOutWhenUnconnected=off
  wires:
  Gain/1 -> Out/1
  Sum1/1 -> Gain/1
  Beta/1 -> Variable Transport Delay/1, Sum1/1
  Alpha/1 -> Variable Transport Delay1/1
  Cos 2*pi/n/1(cos) -> Product/2
  Product/1 -> Sum1/2
  Variable Transport Delay/1 -> Product/1
  Variable Transport Delay1/1 -> Product1/1
  Product1/1 -> Sum1/3
  Sin 2*pi/n/1(sin) -> Product1/2
  T/n/1 -> Divide/1
  Divide/1 -> Variable Transport Delay/2
  [f_pll_c3] -> Divide/2
  T/n1/1 -> Divide1/1
  Divide1/1 -> Variable Transport Delay1/2
  [f_pll_c3] -> Divide1/2

== system MPG_MG_PLL_orig/Voltage Source Inverter 3/CDSC-PLL/DSC16/DSC_alpha ==
  Alpha : Inport
  Beta : Inport  Port=2
  Cos 2*pi/n : Subsystem
  Divide : Product  Inputs=*/
  Divide1 : Product  Inputs=*/
  Gain : Gain  Gain=1/2
  Product : Product
  Product1 : Product
  Sin 2*pi/n : Subsystem
  Sum1 : Sum  Inputs=++-
  T/n : Constant  Value=1/n
  T/n1 : Constant  Value=1/n
  Variable Transport Delay : VariableTransportDelay  VariableDelayType=Variable transport delay  MaximumDelay=10
  Variable Transport Delay1 : VariableTransportDelay  VariableDelayType=Variable transport delay  MaximumDelay=10
  Out : Outport  VectorParamsAs1DForOutWhenUnconnected=off
  wires:
  Sum1/1 -> Gain/1
  Gain/1 -> Out/1
  Sin 2*pi/n/1(sin) -> Product1/2
  Beta/1 -> Variable Transport Delay1/1
  Product1/1 -> Sum1/3
  Variable Transport Delay1/1 -> Product1/1
  Alpha/1 -> Variable Transport Delay/1, Sum1/1
  Variable Transport Delay/1 -> Product/1
  Product/1 -> Sum1/2
  Cos 2*pi/n/1(cos) -> Product/2
  T/n/1 -> Divide/1
  Divide/1 -> Variable Transport Delay/2
  [f_pll_c3] -> Divide/2
  T/n1/1 -> Divide1/1
  Divide1/1 -> Variable Transport Delay1/2
  [f_pll_c3] -> Divide1/2

== system MPG_MG_PLL_orig/Voltage Source Inverter 3/CDSC-PLL/DSC2/DSC_Beta ==
  Alpha : Inport
  Beta : Inport  Port=2
  Cos 2*pi/n : Subsystem
  Divide : Product  Inputs=*/
  Divide1 : Product  Inputs=*/
  Gain : Gain  Gain=1/2
  Product : Product
  Product1 : Product
  Sin 2*pi/n : Subsystem
  Sum1 : Sum  Inputs=+++
  T/n : Constant  Value=1/n
  T/n1 : Constant  Value=1/n
  Variable Transport Delay : VariableTransportDelay  VariableDelayType=Variable transport delay  MaximumDelay=10
  Variable Transport Delay1 : VariableTransportDelay  VariableDelayType=Variable transport delay  MaximumDelay=10
  Out : Outport  VectorParamsAs1DForOutWhenUnconnected=off
  wires:
  Sin 2*pi/n/1(sin) -> Product1/2
  Product1/1 -> Sum1/3
  Variable Transport Delay1/1 -> Product1/1
  Variable Transport Delay/1 -> Product/1
  Product/1 -> Sum1/2
  Cos 2*pi/n/1(cos) -> Product/2
  Alpha/1 -> Variable Transport Delay1/1
  Beta/1 -> Sum1/1, Variable Transport Delay/1
  Sum1/1 -> Gain/1
  Gain/1 -> Out/1
  T/n1/1 -> Divide/1
  Divide/1 -> Variable Transport Delay1/2
  [f_pll_c3] -> Divide/2
  T/n/1 -> Divide1/1
  Divide1/1 -> Variable Transport Delay/2
  [f_pll_c3] -> Divide1/2

== system MPG_MG_PLL_orig/Voltage Source Inverter 3/CDSC-PLL/DSC2/DSC_alpha ==
  Alpha : Inport
  Beta : Inport  Port=2
  Cos 2*pi/n : Subsystem
  Divide : Product  Inputs=*/
  Divide1 : Product  Inputs=*/
  Gain : Gain  Gain=1/2
  Product : Product
  Product1 : Product
  Sin 2*pi/n : Subsystem
  Sum1 : Sum  Inputs=++-
  T/n : Constant  Value=1/n
  T/n. : Constant  Value=1/n
  Variable Transport Delay : VariableTransportDelay  VariableDelayType=Variable transport delay  MaximumDelay=10
  Variable Transport Delay1 : VariableTransportDelay  VariableDelayType=Variable transport delay  MaximumDelay=10
  Out : Outport  VectorParamsAs1DForOutWhenUnconnected=off
  wires:
  Cos 2*pi/n/1(cos) -> Product/2
  Product/1 -> Sum1/2
  Variable Transport Delay/1 -> Product/1
  Alpha/1 -> Variable Transport Delay/1, Sum1/1
  Variable Transport Delay1/1 -> Product1/1
  Product1/1 -> Sum1/3
  Beta/1 -> Variable Transport Delay1/1
  Sin 2*pi/n/1(sin) -> Product1/2
  Gain/1 -> Out/1
  Sum1/1 -> Gain/1
  T/n/1 -> Divide/1
  Divide/1 -> Variable Transport Delay/2
  [f_pll_c3] -> Divide/2
  Divide1/1 -> Variable Transport Delay1/2
  T/n./1 -> Divide1/1
  [f_pll_c3] -> Divide1/2

== system MPG_MG_PLL_orig/Voltage Source Inverter 3/CDSC-PLL/DSC4/DSC_Beta ==
  Alpha : Inport
  Beta : Inport  Port=2
  Cos 2*pi/n : Subsystem
  Divide : Product  Inputs=*/
  Divide1 : Product  Inputs=*/
  Gain : Gain  Gain=1/2
  Product : Product
  Product1 : Product
  Sin 2*pi/n : Subsystem
  Sum1 : Sum  Inputs=+++
  T/n : Constant  Value=1/n
  T/n1 : Constant  Value=1/n
  Variable Transport Delay : VariableTransportDelay  VariableDelayType=Variable transport delay  MaximumDelay=10
  Variable Transport Delay1 : VariableTransportDelay  VariableDelayType=Variable transport delay  MaximumDelay=10
  Out : Outport  VectorParamsAs1DForOutWhenUnconnected=off
  wires:
  Gain/1 -> Out/1
  Sum1/1 -> Gain/1
  Beta/1 -> Variable Transport Delay/1, Sum1/1
  Alpha/1 -> Variable Transport Delay1/1
  Cos 2*pi/n/1(cos) -> Product/2
  Product/1 -> Sum1/2
  Variable Transport Delay/1 -> Product/1
  Variable Transport Delay1/1 -> Product1/1
  Product1/1 -> Sum1/3
  Sin 2*pi/n/1(sin) -> Product1/2
  T/n/1 -> Divide/1
  Divide/1 -> Variable Transport Delay/2
  [f_pll_c3] -> Divide/2
  T/n1/1 -> Divide1/1
  Divide1/1 -> Variable Transport Delay1/2
  [f_pll_c3] -> Divide1/2

== system MPG_MG_PLL_orig/Voltage Source Inverter 3/CDSC-PLL/DSC4/DSC_alpha ==
  Alpha : Inport
  Beta : Inport  Port=2
  Cos 2*pi/n : Subsystem
  Divide : Product  Inputs=*/
  Divide1 : Product  Inputs=*/
  Gain : Gain  Gain=1/2
  Product : Product
  Product1 : Product
  Sin 2*pi/n : Subsystem
  Sum1 : Sum  Inputs=++-
  T/n : Constant  Value=1/n
  T/n1 : Constant  Value=1/n
  Variable Transport Delay : VariableTransportDelay  VariableDelayType=Variable transport delay  MaximumDelay=10
  Variable Transport Delay1 : VariableTransportDelay  VariableDelayType=Variable transport delay  MaximumDelay=10
  Out : Outport  VectorParamsAs1DForOutWhenUnconnected=off
  wires:
  Sum1/1 -> Gain/1
  Gain/1 -> Out/1
  Sin 2*pi/n/1(sin) -> Product1/2
  Beta/1 -> Variable Transport Delay1/1
  Product1/1 -> Sum1/3
  Variable Transport Delay1/1 -> Product1/1
  Alpha/1 -> Variable Transport Delay/1, Sum1/1
  Variable Transport Delay/1 -> Product/1
  Product/1 -> Sum1/2
  Cos 2*pi/n/1(cos) -> Product/2
  T/n1/1 -> Divide/1
  Divide/1 -> Variable Transport Delay1/2
  [f_pll_c3] -> Divide/2
  T/n/1 -> Divide1/1
  Divide1/1 -> Variable Transport Delay/2
  [f_pll_c3] -> Divide1/2

== system MPG_MG_PLL_orig/Voltage Source Inverter 3/CDSC-PLL/DSC8/DSC_Beta ==
  Alpha : Inport
  Beta : Inport  Port=2
  Cos 2*pi/n : Subsystem
  Divide : Product  Inputs=*/
  Divide1 : Product  Inputs=*/
  Gain : Gain  Gain=1/2
  Product : Product
  Product1 : Product
  Sin 2*pi/n : Subsystem
  Sum1 : Sum  Inputs=+++
  T/n : Constant  Value=1/n
  T/n1 : Constant  Value=1/n
  Variable Transport Delay : VariableTransportDelay  VariableDelayType=Variable transport delay  MaximumDelay=10
  Variable Transport Delay1 : VariableTransportDelay  VariableDelayType=Variable transport delay  MaximumDelay=10
  Out : Outport  VectorParamsAs1DForOutWhenUnconnected=off
  wires:
  Sin 2*pi/n/1(sin) -> Product1/2
  Product1/1 -> Sum1/3
  Variable Transport Delay1/1 -> Product1/1
  Variable Transport Delay/1 -> Product/1
  Product/1 -> Sum1/2
  Cos 2*pi/n/1(cos) -> Product/2
  Alpha/1 -> Variable Transport Delay1/1
  Beta/1 -> Sum1/1, Variable Transport Delay/1
  Sum1/1 -> Gain/1
  Gain/1 -> Out/1
  T/n/1 -> Divide/1
  Divide/1 -> Variable Transport Delay/2
  [f_pll_c3] -> Divide/2
  T/n1/1 -> Divide1/1
  Divide1/1 -> Variable Transport Delay1/2
  [f_pll_c3] -> Divide1/2

== system MPG_MG_PLL_orig/Voltage Source Inverter 3/CDSC-PLL/DSC8/DSC_alpha ==
  Alpha : Inport
  Beta : Inport  Port=2
  Cos 2*pi/n : Subsystem
  Divide : Product  Inputs=*/
  Divide1 : Product  Inputs=*/
  Gain : Gain  Gain=1/2
  Product : Product
  Product1 : Product
  Sin 2*pi/n : Subsystem
  Sum1 : Sum  Inputs=++-
  T/n : Constant  Value=1/n
  T/n1 : Constant  Value=1/n
  Variable Transport Delay : VariableTransportDelay  VariableDelayType=Variable transport delay  MaximumDelay=10
  Variable Transport Delay1 : VariableTransportDelay  VariableDelayType=Variable transport delay  MaximumDelay=10
  Out : Outport  VectorParamsAs1DForOutWhenUnconnected=off
  wires:
  Cos 2*pi/n/1(cos) -> Product/2
  Product/1 -> Sum1/2
  Variable Transport Delay/1 -> Product/1
  Alpha/1 -> Variable Transport Delay/1, Sum1/1
  Variable Transport Delay1/1 -> Product1/1
  Product1/1 -> Sum1/3
  Beta/1 -> Variable Transport Delay1/1
  Sin 2*pi/n/1(sin) -> Product1/2
  Gain/1 -> Out/1
  Sum1/1 -> Gain/1
  T/n/1 -> Divide/1
  Divide/1 -> Variable Transport Delay/2
  [f_pll_c3] -> Divide/2
  T/n1/1 -> Divide1/1
  Divide1/1 -> Variable Transport Delay1/2
  [f_pll_c3] -> Divide1/2

== system MPG_MG_PLL_orig/Voltage Source Inverter 3/CDSC-PLL/SRF-PLL1/Al_Be_0 to dq0 ==
  Al_Be_0 : Inport
  wt : Inport  Port=2
  Fcn : Fcn  Expr=u[1]*cos(u[4]) + u[2]*sin(u[4])
  Fcn1 : Fcn  Expr=-u[1]*sin(u[4]) + u[2]*cos(u[4])
  Fcn2 : Fcn  Expr=u[3]
  Mux1 : Mux  Inputs=[3 1]
  Mux2 : Mux  Inputs=3
  dq0 : Outport  VectorParamsAs1DForOutWhenUnconnected=off
  wires:
  Mux1/1 -> Fcn/1, Fcn2/1, Fcn1/1
  Fcn1/1 -> Mux2/2
  wt/1 -> Mux1/2
  Mux2/1 -> dq0/1
  Al_Be_0/1 -> Mux1/1
  Fcn2/1 -> Mux2/3
  Fcn/1 -> Mux2/1

== system MPG_MG_PLL_orig/Voltage Source Inverter 4/CDSC-PLL/DSC16/DSC_Beta ==
  Alpha : Inport
  Beta : Inport  Port=2
  Cos 2*pi/n : Subsystem
  Divide : Product  Inputs=*/
  Divide1 : Product  Inputs=*/
  Gain : Gain  Gain=1/2
  Product : Product
  Product1 : Product
  Sin 2*pi/n : Subsystem
  Sum1 : Sum  Inputs=+++
  T/n : Constant  Value=1/n
  T/n1 : Constant  Value=1/n
  Variable Transport Delay : VariableTransportDelay  VariableDelayType=Variable transport delay  MaximumDelay=10
  Variable Transport Delay1 : VariableTransportDelay  VariableDelayType=Variable transport delay  MaximumDelay=10
  Out : Outport  VectorParamsAs1DForOutWhenUnconnected=off
  wires:
  Gain/1 -> Out/1
  Sum1/1 -> Gain/1
  Beta/1 -> Variable Transport Delay/1, Sum1/1
  Alpha/1 -> Variable Transport Delay1/1
  Cos 2*pi/n/1(cos) -> Product/2
  Product/1 -> Sum1/2
  Variable Transport Delay/1 -> Product/1
  Variable Transport Delay1/1 -> Product1/1
  Product1/1 -> Sum1/3
  Sin 2*pi/n/1(sin) -> Product1/2
  T/n/1 -> Divide/1
  Divide/1 -> Variable Transport Delay/2
  [f_pll_c3] -> Divide/2
  T/n1/1 -> Divide1/1
  Divide1/1 -> Variable Transport Delay1/2
  [f_pll_c3] -> Divide1/2

== system MPG_MG_PLL_orig/Voltage Source Inverter 4/CDSC-PLL/DSC16/DSC_alpha ==
  Alpha : Inport
  Beta : Inport  Port=2
  Cos 2*pi/n : Subsystem
  Divide : Product  Inputs=*/
  Divide1 : Product  Inputs=*/
  Gain : Gain  Gain=1/2
  Product : Product
  Product1 : Product
  Sin 2*pi/n : Subsystem
  Sum1 : Sum  Inputs=++-
  T/n : Constant  Value=1/n
  T/n1 : Constant  Value=1/n
  Variable Transport Delay : VariableTransportDelay  VariableDelayType=Variable transport delay  MaximumDelay=10
  Variable Transport Delay1 : VariableTransportDelay  VariableDelayType=Variable transport delay  MaximumDelay=10
  Out : Outport  VectorParamsAs1DForOutWhenUnconnected=off
  wires:
  Sum1/1 -> Gain/1
  Gain/1 -> Out/1
  Sin 2*pi/n/1(sin) -> Product1/2
  Beta/1 -> Variable Transport Delay1/1
  Product1/1 -> Sum1/3
  Variable Transport Delay1/1 -> Product1/1
  Alpha/1 -> Variable Transport Delay/1, Sum1/1
  Variable Transport Delay/1 -> Product/1
  Product/1 -> Sum1/2
  Cos 2*pi/n/1(cos) -> Product/2
  T/n/1 -> Divide/1
  Divide/1 -> Variable Transport Delay/2
  [f_pll_c3] -> Divide/2
  T/n1/1 -> Divide1/1
  Divide1/1 -> Variable Transport Delay1/2
  [f_pll_c3] -> Divide1/2

== system MPG_MG_PLL_orig/Voltage Source Inverter 4/CDSC-PLL/DSC2/DSC_Beta ==
  Alpha : Inport
  Beta : Inport  Port=2
  Cos 2*pi/n : Subsystem
  Divide : Product  Inputs=*/
  Divide1 : Product  Inputs=*/
  Gain : Gain  Gain=1/2
  Product : Product
  Product1 : Product
  Sin 2*pi/n : Subsystem
  Sum1 : Sum  Inputs=+++
  T/n : Constant  Value=1/n
  T/n1 : Constant  Value=1/n
  Variable Transport Delay : VariableTransportDelay  VariableDelayType=Variable transport delay  MaximumDelay=10
  Variable Transport Delay1 : VariableTransportDelay  VariableDelayType=Variable transport delay  MaximumDelay=10
  Out : Outport  VectorParamsAs1DForOutWhenUnconnected=off
  wires:
  Sin 2*pi/n/1(sin) -> Product1/2
  Product1/1 -> Sum1/3
  Variable Transport Delay1/1 -> Product1/1
  Variable Transport Delay/1 -> Product/1
  Product/1 -> Sum1/2
  Cos 2*pi/n/1(cos) -> Product/2
  Alpha/1 -> Variable Transport Delay1/1
  Beta/1 -> Sum1/1, Variable Transport Delay/1
  Sum1/1 -> Gain/1
  Gain/1 -> Out/1
  T/n1/1 -> Divide/1
  Divide/1 -> Variable Transport Delay1/2
  [f_pll_c3] -> Divide/2
  T/n/1 -> Divide1/1
  Divide1/1 -> Variable Transport Delay/2
  [f_pll_c3] -> Divide1/2

== system MPG_MG_PLL_orig/Voltage Source Inverter 4/CDSC-PLL/DSC2/DSC_alpha ==
  Alpha : Inport
  Beta : Inport  Port=2
  Cos 2*pi/n : Subsystem
  Divide : Product  Inputs=*/
  Divide1 : Product  Inputs=*/
  Gain : Gain  Gain=1/2
  Product : Product
  Product1 : Product
  Sin 2*pi/n : Subsystem
  Sum1 : Sum  Inputs=++-
  T/n : Constant  Value=1/n
  T/n. : Constant  Value=1/n
  Variable Transport Delay : VariableTransportDelay  VariableDelayType=Variable transport delay  MaximumDelay=10
  Variable Transport Delay1 : VariableTransportDelay  VariableDelayType=Variable transport delay  MaximumDelay=10
  Out : Outport  VectorParamsAs1DForOutWhenUnconnected=off
  wires:
  Cos 2*pi/n/1(cos) -> Product/2
  Product/1 -> Sum1/2
  Variable Transport Delay/1 -> Product/1
  Alpha/1 -> Variable Transport Delay/1, Sum1/1
  Variable Transport Delay1/1 -> Product1/1
  Product1/1 -> Sum1/3
  Beta/1 -> Variable Transport Delay1/1
  Sin 2*pi/n/1(sin) -> Product1/2
  Gain/1 -> Out/1
  Sum1/1 -> Gain/1
  T/n/1 -> Divide/1
  Divide/1 -> Variable Transport Delay/2
  [f_pll_c3] -> Divide/2
  Divide1/1 -> Variable Transport Delay1/2
  T/n./1 -> Divide1/1
  [f_pll_c3] -> Divide1/2
